simulink model "X15_PIO"  (R2026a)
settings: Solver=VariableStepAuto  StopTime=90
values from neighbouring files (symbols this model uses):
  R = 15    [draw_figure7.m]    (also in draw_figure7_chirp.m; x15_pio_figures.m; x15_pio_figures_updated.m)
undefined symbols (not defined in the file or in its folder): Kact, Kp, thau, Tkick
settings Model: Creator=t0900  LastModifiedBy=t0900

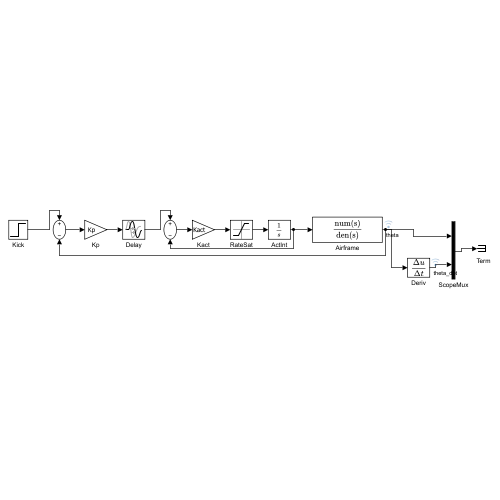
[thumbnail: Simulink's stored preview of the top-level diagram]
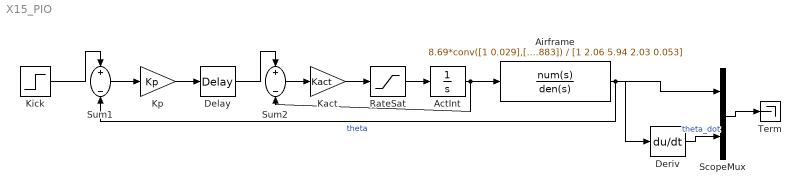
== system X15_PIO ==
  ActInt : Integrator
  Airframe : TransferFcn  Numerator=8.69*conv([1 0.029],[1 0.883])  Denominator=[1 2.06 5.94 2.03 0.053]
  Delay : TransportDelay  DelayTime=thau
  Deriv : Derivative
  Kact : Gain  Gain=Kact
  Kick : Step  Time=Tkick  InitialValue=Akick  FinalValue=0  SampleTime=0
  Kp : Gain  Gain=Kp
  RateSat : Saturate  UpperLimit=R  LowerLimit=-R
  ScopeMux : Mux  Inputs=2
  Sum1 : Sum  Inputs=+-
  Sum2 : Sum  Inputs=+-
  Term : Terminator
  wires:
  Kick/1 -> Sum1/1
  Sum1/1 -> Kp/1
  Kp/1 -> Delay/1
  Delay/1 -> Sum2/1
  Sum2/1 -> Kact/1
  Kact/1 -> RateSat/1
  RateSat/1 -> ActInt/1
  ActInt/1 -> Airframe/1, Sum2/2
  Airframe/1 -> Sum1/2, Deriv/1, ScopeMux/1  "theta"
  Deriv/1 -> ScopeMux/2  "theta_dot"
  ScopeMux/1 -> Term/1
